simulink model "Group_11_Assignment_3_Task_D_Simulink_model"  (R2019b)
settings: Solver=FixedStepDiscrete  StartTime=0.0  StopTime=100  FixedStep=h  RelTol=1e-3  EnableMultiTasking=on
values from neighbouring files (symbols this model uses):
  Add = p.A    [Assignment_2_Group_11_code.m]    (also in Group_11_Assignment_3_code.m)
  Bdd = p.B    [Assignment_2_Group_11_code.m]    (also in Group_11_Assignment_3_code.m)
  Cdd = p.C    [Group_11_Assignment_3_code.m]
  h = 0.001    [Group_11_Assignment_3_code.m]
  L_I = L_LQ(:,6)    [Group_11_Assignment_3_code.m]
  L_P = L_LQ(:,1:5)    [Group_11_Assignment_3_code.m]
  Qn = R1    [Group_11_Assignment_3_code.m]
  Rn = R2    [Group_11_Assignment_3_code.m]
undefined symbols (not defined in the file or in its folder): DiscIntNeverNeededParam, K
settings Model: Creator=tw  LastModifiedBy=Mani
settings DataIOCC: LimitDataPoints=on  MaxDataPoints=1000000  SaveFormat=Array  SignalLoggingSaveFormat=ModelDataLogs  ReturnWorkspaceOutputs=off
settings OptimizationCC: ExpressionDepthLimit=2147483647  InitFltsAndDblsToZero=on  LifeSpan=inf
settings DebuggingCC: SaveWithParameterizedLinksMsg=none  UnderspecifiedInitializationDetection=Classic  MergeDetectMultiDrivingBlocksExec=none  SolverPrmCheckMsg=warning  FcnCallInpInsideContextMsg=warning  StateNameClashWarn=warning  SFUnexpectedBacktrackingDiag=warning  SFNoUnconditionalDefaultTransitionDiag=warning  SFExecutionAtInitializationDiag=none  ArithmeticOperatorsInVariantConditions=warning
settings HardwareCC: ProdBitPerPointer=32  ProdBitPerSizeT=32  ProdBitPerPtrDiffT=32  ProdLargestAtomicFloat=None  ProdIntDivRoundTo=Undefined  ProdEndianess=Unspecified  ProdWordSize=32  ProdHWDeviceType=32-bit Generic
settings ModelReferenceCC: PropagateSignalLabelsOutOfModel=off
settings SFSimCC: SimUseLocalCustomCode=off  CustomCodeUndefinedFunction=UseInterfaceOnly
settings RTWCC: RTWUseLocalCustomCode=off
settings CodeAppCC: StateflowObjectComments=on
settings GRTTargetCC: TargetFcnLib=ansi_tfl_tmw.mat  TargetLangStandard=C89/C90 (ANSI)  CombineOutputUpdateFcns=off  GRTInterface=on
settings ConfigComp: CovMetricSettings=dw  CovHtmlReporting=on  CovSaveCumulativeToWorkspaceVar=on  CovSaveSingleToWorkspaceVar=on  CovExternalEMLEnable=off

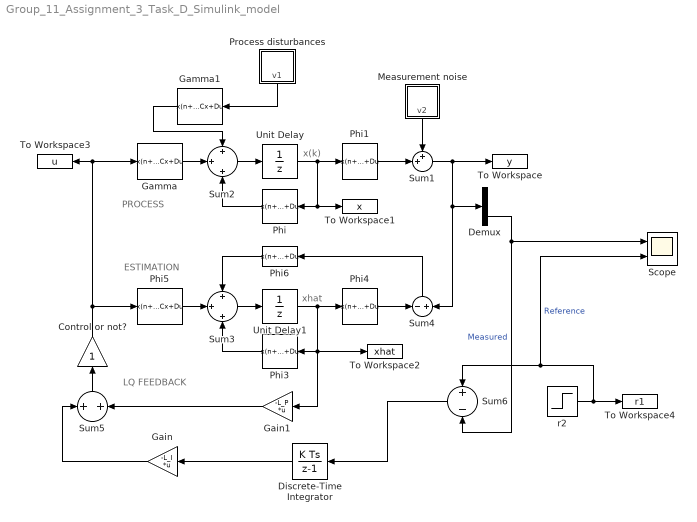
== system Group_11_Assignment_3_Task_D_Simulink_model ==
  note: x(k)
  note: xhat
  note: PROCESS
  note: LQ FEEDBACK
  note: ESTIMATION
  Control or not? : Gain
  Demux : Demux  Outputs=2
  Discrete-Time Integrator : DiscreteIntegrator  SampleTime=-1  ICPrevOutput=DiscIntNeverNeededParam  ICPrevScaledInput=DiscIntNeverNeededParam
  Gain : Gain  Gain=-L_I  Multiplication=Matrix(K*u)
  Gain1 : Gain  Gain=-L_P  Multiplication=Matrix(K*u)
  Gamma : DiscreteStateSpace  A=[]  B=[]  C=[]  D=Bdd  SampleTime=-1  mask(Vector gain){}
      mask Display: disp('Bd')
  Gamma1 : DiscreteStateSpace  A=[]  B=[]  C=[]  D=Bdd  SampleTime=-1  mask(Vector gain){}
      mask Display: disp('Bd')
  Measurement noise : Subsystem
  Phi : DiscreteStateSpace  A=[]  B=[]  C=[]  D=Add  SampleTime=-1  mask(Vector gain){}
      mask Display: disp('Ad')
  Phi1 : DiscreteStateSpace  A=[]  B=[]  C=[]  D=Cdd  SampleTime=-1  mask(Vector gain){}
      mask Display: disp('C')
  Phi3 : DiscreteStateSpace  A=[]  B=[]  C=[]  D=Add  SampleTime=-1  mask(Vector gain){}
      mask Display: disp('Ad')
  Phi4 : DiscreteStateSpace  A=[]  B=[]  C=[]  D=Cdd  SampleTime=-1  mask(Vector gain){}
      mask Display: disp('C')
  Phi5 : DiscreteStateSpace  A=[]  B=[]  C=[]  D=Bdd  SampleTime=-1  mask(Vector gain){}
      mask Display: disp('Bd')
  Phi6 : DiscreteStateSpace  A=[]  B=[]  C=[]  D=K  SampleTime=-1  mask(Vector gain){}
      mask Display: disp('K')
  Process disturbances : Subsystem
  "Scope " : Scope  NumInputPorts=2
  Sum1 : Sum  Inputs=++|
  Sum2 : Sum  Inputs=+|+|+
  Sum3 : Sum  Inputs=+|+|+
  Sum4 : Sum  Inputs=-|+
  Sum5 : Sum  Inputs=+|+
  Sum6 : Sum  Inputs=+-
  To Workspace : ToWorkspace  VariableName=y  SampleTime=-1
  To Workspace1 : ToWorkspace  VariableName=x  SampleTime=-1
  To Workspace2 : ToWorkspace  VariableName=xhat  SampleTime=-1
  To Workspace3 : ToWorkspace  VariableName=u  SampleTime=-1
  To Workspace4 : ToWorkspace  VariableName=r1  SampleTime=-1
  Unit Delay : UnitDelay  SampleTime=-1  HasFrameUpgradeWarning=on
  Unit Delay1 : UnitDelay  SampleTime=-1  HasFrameUpgradeWarning=on
  r2 : Step  Time=10  Before=10  After=100  SampleTime=h
  wires:
  Sum2/1 -> Unit Delay/1
  Unit Delay/1 -> Phi1/1, Phi/1, To Workspace1/1
  Phi1/1 -> Sum1/2
  Sum1/1 -> Demux/1, Sum4/2, To Workspace/1
  Measurement noise/1(v2) -> Sum1/1
  Process disturbances/1(v1) -> Gamma1/1
  Gamma/1 -> Sum2/2
  Phi/1 -> Sum2/3
  Sum3/1 -> Unit Delay1/1
  Unit Delay1/1 -> Phi4/1, Gain1/1, Phi3/1, To Workspace2/1
  Phi5/1 -> Sum3/2
  Phi3/1 -> Sum3/3
  Phi4/1 -> Sum4/1
  Sum4/1 -> Phi6/1
  Phi6/1 -> Sum3/1
  Sum5/1 -> Control or not?/1
  Control or not?/1 -> Phi5/1, Gamma/1, To Workspace3/1
  Gamma1/1 -> Sum2/1
  Gain/1 -> Sum5/1
  Discrete-Time Integrator/1 -> Gain/1
  Sum6/1 -> Discrete-Time Integrator/1
  Demux/2 -> "Scope "/1, Sum6/2  "Measured"
  Gain1/1 -> Sum5/2
  r2/1 -> "Scope "/2, Sum6/1, To Workspace4/1  "Reference"

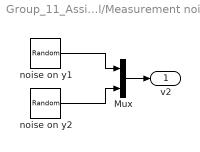
== system Group_11_Assignment_3_Task_D_Simulink_model/Measurement noise ==
  Mux : Mux  Inputs=2
  noise on y1 : RandomNumber  Variance=Rn(1,1)  Seed=5  SampleTime=h
  noise on y2 : RandomNumber  Variance=Rn(2,2)  Seed=4  SampleTime=h
  v2 : Outport
  wires:
  noise on y1/1 -> Mux/1
  noise on y2/1 -> Mux/2
  Mux/1 -> v2/1

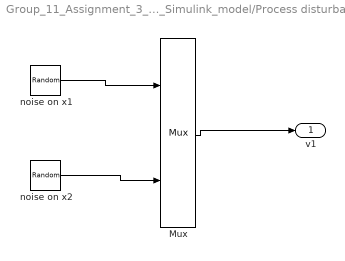
== system Group_11_Assignment_3_Task_D_Simulink_model/Process disturbances ==
  Mux : Mux  Inputs=2
  noise on x1 : RandomNumber  Variance=Qn(1,1)  Seed=3  SampleTime=h
  noise on x2 : RandomNumber  Variance=Qn(2,2)  Seed=2  SampleTime=h
  v1 : Outport
  wires:
  noise on x1/1 -> Mux/1
  Mux/1 -> v1/1
  noise on x2/1 -> Mux/2
